simulink model "P702_NI_SoftECU"  (R2019a)
settings: Solver=ode1  StartTime=0.0  StopTime=Inf  FixedStep=0.001  RelTol=1e-3  EnableMultiTasking=on
PreLoadFcn:
  | run '.\VeriStand_BlockSet\NIVeriStandAddPaths.m'
undefined symbols (not defined in the file or in its folder): magnitude
libraries: simulink x83, simulink_extras x1
(part 75 of 76)

== system P702_NI_SoftECU/Output/Subsystem2/CAN_Signal/GWM/Other_GWMTx/Power_Liftgate_Stat_FD1 ==
  DrLckCnt_No_ActlTgate : Constant  Value=0
  DrTGate_D_Rq : Constant  Value=0
  DrTgateChime2_D_Rq : Constant  Value=0
  Power_Liftgate_Mode_Stt : Constant  Value=0
  PwLftgtIntSw_B_Stat : Constant  Value=0
  bus_creator : BusCreator  Inputs=5
  out_port : Outport
  wires:
  bus_creator/1 -> out_port/1  "Subsystem2"
  DrLckCnt_No_ActlTgate/1 -> bus_creator/1  "DrLckCnt_No_ActlTgate"
  DrTGate_D_Rq/1 -> bus_creator/2  "DrTGate_D_Rq"
  DrTgateChime2_D_Rq/1 -> bus_creator/3  "DrTgateChime2_D_Rq"
  Power_Liftgate_Mode_Stt/1 -> bus_creator/4  "Power_Liftgate_Mode_Stt"
  PwLftgtIntSw_B_Stat/1 -> bus_creator/5  "PwLftgtIntSw_B_Stat"

== system P702_NI_SoftECU/Output/Subsystem2/CAN_Signal/GWM/Other_GWMTx/PreCond_Hev_Data1_FD1 ==
  ChrgStat_D2_Dsply : Constant  Value=0
  bus_creator : BusCreator  Inputs=1
  out_port : Outport
  wires:
  bus_creator/1 -> out_port/1  "Subsystem2"
  ChrgStat_D2_Dsply/1 -> bus_creator/1  "ChrgStat_D2_Dsply"

== system P702_NI_SoftECU/Output/Subsystem2/CAN_Signal/GWM/Other_GWMTx/PreCond_Hev_Data2_FD1 ==
  BattTracClntFlw_Pc_Rq : Constant  Value=0
  BattTrac_I_EstVsc : Constant  Value=0
  DrvCondTpRrDefrs_B_Rq : Constant  Value=0
  HtrnAin_UHi_Actl : Constant  Value=0
  HtrnHvilOpen_B_Actl : Constant  Value=0
  HtrnMil_D_Rq : Constant  Value=0
  HtrnOvrTeLamp_B_Dsply : Constant  Value=0
  HtrnSrvcRqd_B_Dsply : Constant  Value=0
  PreCondActv_B_Actl : Constant  Value=0
  PtWakeupDeltaT_T_Rq : Constant  Value=0
  bus_creator : BusCreator  Inputs=10
  out_port : Outport
  wires:
  bus_creator/1 -> out_port/1  "Subsystem2"
  BattTracClntFlw_Pc_Rq/1 -> bus_creator/1  "BattTracClntFlw_Pc_Rq"
  BattTrac_I_EstVsc/1 -> bus_creator/2  "BattTrac_I_EstVsc"
  DrvCondTpRrDefrs_B_Rq/1 -> bus_creator/3  "DrvCondTpRrDefrs_B_Rq"
  HtrnAin_UHi_Actl/1 -> bus_creator/4  "HtrnAin_UHi_Actl"
  HtrnHvilOpen_B_Actl/1 -> bus_creator/5  "HtrnHvilOpen_B_Actl"
  HtrnMil_D_Rq/1 -> bus_creator/6  "HtrnMil_D_Rq"
  HtrnOvrTeLamp_B_Dsply/1 -> bus_creator/7  "HtrnOvrTeLamp_B_Dsply"
  HtrnSrvcRqd_B_Dsply/1 -> bus_creator/8  "HtrnSrvcRqd_B_Dsply"
  PreCondActv_B_Actl/1 -> bus_creator/9  "PreCondActv_B_Actl"
  PtWakeupDeltaT_T_Rq/1 -> bus_creator/10  "PtWakeupDeltaT_T_Rq"

== system P702_NI_SoftECU/Output/Subsystem2/CAN_Signal/GWM/Other_GWMTx/Suspension_Data_FD1 ==
  SuspClkSync_No_Rq : Constant  Value=0
  SuspFrntRight_L_Actl : Constant  Value=0
  SuspFrnt_L_Actl : Constant  Value=0
  SuspFrnt_L_Prev : Constant  Value=0
  SuspRearRight_L_Actl : Constant  Value=0
  SuspRear_L_Actl : Constant  Value=0
  SuspRear_L_Prev : Constant  Value=0
  bus_creator : BusCreator  Inputs=7
  out_port : Outport
  wires:
  bus_creator/1 -> out_port/1  "Subsystem2"
  SuspClkSync_No_Rq/1 -> bus_creator/1  "SuspClkSync_No_Rq"
  SuspFrntRight_L_Actl/1 -> bus_creator/2  "SuspFrntRight_L_Actl"
  SuspFrnt_L_Actl/1 -> bus_creator/3  "SuspFrnt_L_Actl"
  SuspFrnt_L_Prev/1 -> bus_creator/4  "SuspFrnt_L_Prev"
  SuspRearRight_L_Actl/1 -> bus_creator/5  "SuspRearRight_L_Actl"
  SuspRear_L_Actl/1 -> bus_creator/6  "SuspRear_L_Actl"
  SuspRear_L_Prev/1 -> bus_creator/7  "SuspRear_L_Prev"

== system P702_NI_SoftECU/Output/Subsystem2/CAN_Signal/GWM/Other_GWMTx/TesterPhysicalResGWM_FD1 ==
  TesterPhysicalResGWM_F1 : Constant  Value=0
  bus_creator : BusCreator  Inputs=1
  out_port : Outport
  wires:
  bus_creator/1 -> out_port/1  "Subsystem2"
  TesterPhysicalResGWM_F1/1 -> bus_creator/1  "TesterPhysicalResGWM_F1"

== system P702_NI_SoftECU/Output/Subsystem2/CAN_Signal/GWM/Other_GWMTx/TrailerAid_Data_FD1 ==
  TrlBrkInitOut_D_Rq : Constant  Value=0
  TrlrAidEnbl_D_Rq : Constant  Value=0
  TrlrAidSetup_D_Rq : Constant  Value=0
  TrlrAnOffstDir_D_Mem : Constant  Value=0
  TrlrAnOffst_An_Mem : Constant  Value=0
  TrlrAxleToBmpr_L_Actl : Constant  Value=0
  TrlrBallToBmpr_L_Actl : Constant  Value=0
  TrlrId_No_Actl : Constant  Value=0
  TrlrRvrseCancl_B_Rq : Constant  Value=0
  TrlrTrgtOffst_L_Actl : Constant  Value=0
  TrlrTrgtPtrnId_No_Mem : Constant  Value=0
  TrlrTrgtToBmpr_L_Actl : Constant  Value=0
  bus_creator : BusCreator  Inputs=12
  out_port : Outport
  wires:
  bus_creator/1 -> out_port/1  "Subsystem2"
  TrlBrkInitOut_D_Rq/1 -> bus_creator/1  "TrlBrkInitOut_D_Rq"
  TrlrAidEnbl_D_Rq/1 -> bus_creator/2  "TrlrAidEnbl_D_Rq"
  TrlrAidSetup_D_Rq/1 -> bus_creator/3  "TrlrAidSetup_D_Rq"
  TrlrAnOffstDir_D_Mem/1 -> bus_creator/4  "TrlrAnOffstDir_D_Mem"
  TrlrAnOffst_An_Mem/1 -> bus_creator/5  "TrlrAnOffst_An_Mem"
  TrlrAxleToBmpr_L_Actl/1 -> bus_creator/6  "TrlrAxleToBmpr_L_Actl"
  TrlrBallToBmpr_L_Actl/1 -> bus_creator/7  "TrlrBallToBmpr_L_Actl"
  TrlrId_No_Actl/1 -> bus_creator/8  "TrlrId_No_Actl"
  TrlrRvrseCancl_B_Rq/1 -> bus_creator/9  "TrlrRvrseCancl_B_Rq"
  TrlrTrgtOffst_L_Actl/1 -> bus_creator/10  "TrlrTrgtOffst_L_Actl"
  TrlrTrgtPtrnId_No_Mem/1 -> bus_creator/11  "TrlrTrgtPtrnId_No_Mem"
  TrlrTrgtToBmpr_L_Actl/1 -> bus_creator/12  "TrlrTrgtToBmpr_L_Actl"

== system P702_NI_SoftECU/Output/Subsystem2/CAN_Signal/GWM/Other_GWMTx/TrailerAid_Stat1_FD1 ==
  TrlrSnsId_No_Actl : Constant  Value=0
  bus_creator : BusCreator  Inputs=1
  out_port : Outport
  wires:
  bus_creator/1 -> out_port/1  "Subsystem2"
  TrlrSnsId_No_Actl/1 -> bus_creator/1  "TrlrSnsId_No_Actl"

== system P702_NI_SoftECU/Output/Subsystem2/CAN_Signal/GWM/Other_GWMTx/TrailerAid_Stat2_FD1 ==
  TrlrHitYaw_AnRate_Actl : Constant  Value=0
  TrlrHitchYaw_An_Actl : Constant  Value=0
  TrlrHitchYaw_D_Stat : Constant  Value=0
  TrlrYawWActl_D_Qf : Constant  Value=0
  TrlrYaw_W_Actl : Constant  Value=0
  bus_creator : BusCreator  Inputs=5
  out_port : Outport
  wires:
  bus_creator/1 -> out_port/1  "Subsystem2"
  TrlrHitYaw_AnRate_Actl/1 -> bus_creator/1  "TrlrHitYaw_AnRate_Actl"
  TrlrHitchYaw_An_Actl/1 -> bus_creator/2  "TrlrHitchYaw_An_Actl"
  TrlrHitchYaw_D_Stat/1 -> bus_creator/3  "TrlrHitchYaw_D_Stat"
  TrlrYawWActl_D_Qf/1 -> bus_creator/4  "TrlrYawWActl_D_Qf"
  TrlrYaw_W_Actl/1 -> bus_creator/5  "TrlrYaw_W_Actl"

== system P702_NI_SoftECU/Output/Subsystem2/CAN_Signal/GWM/Other_GWMTx/TrailerBrakeInfo_FD1 ==
  StopLamp_B_RqTrlrBrk : Constant  Value=0
  TrlBrkInitOut_D_Stat : Constant  Value=0
  TrlrBrkActCirct_B_Falt : Constant  Value=0
  TrlrBrkActCnnct_B_Actl : Constant  Value=0
  TrlrBrkCtl_B_Falt : Constant  Value=0
  TrlrBrkDcnnt_B_Actl : Constant  Value=0
  TrlrBrkDsply_B_Rq : Constant  Value=0
  TrlrBrkGain_No_Actl : Constant  Value=0
  TrlrBrkMde_D_Actl : Constant  Value=0
  TrlrBrkOut_No_Dsply : Constant  Value=0
  bus_creator : BusCreator  Inputs=10
  out_port : Outport
  wires:
  bus_creator/1 -> out_port/1  "Subsystem2"
  StopLamp_B_RqTrlrBrk/1 -> bus_creator/1  "StopLamp_B_RqTrlrBrk"
  TrlBrkInitOut_D_Stat/1 -> bus_creator/2  "TrlBrkInitOut_D_Stat"
  TrlrBrkActCirct_B_Falt/1 -> bus_creator/3  "TrlrBrkActCirct_B_Falt"
  TrlrBrkActCnnct_B_Actl/1 -> bus_creator/4  "TrlrBrkActCnnct_B_Actl"
  TrlrBrkCtl_B_Falt/1 -> bus_creator/5  "TrlrBrkCtl_B_Falt"
  TrlrBrkDcnnt_B_Actl/1 -> bus_creator/6  "TrlrBrkDcnnt_B_Actl"
  TrlrBrkDsply_B_Rq/1 -> bus_creator/7  "TrlrBrkDsply_B_Rq"
  TrlrBrkGain_No_Actl/1 -> bus_creator/8  "TrlrBrkGain_No_Actl"
  TrlrBrkMde_D_Actl/1 -> bus_creator/9  "TrlrBrkMde_D_Actl"
  TrlrBrkOut_No_Dsply/1 -> bus_creator/10  "TrlrBrkOut_No_Dsply"

== system P702_NI_SoftECU/Output/Subsystem2/CAN_Signal/GWM/Other_GWMTx/TrailerInfo_2_FD1 ==
  TrlrAidAn_URate_Actl : Constant  Value=0
  TrlrAidAn_U_Actl : Constant  Value=0
  TrlrAidCtl_U_RqDrv : Constant  Value=0
  TrlrAidSwtch_D_RqDrv : Constant  Value=0
  bus_creator : BusCreator  Inputs=4
  out_port : Outport
  wires:
  bus_creator/1 -> out_port/1  "Subsystem2"
  TrlrAidAn_URate_Actl/1 -> bus_creator/1  "TrlrAidAn_URate_Actl"
  TrlrAidAn_U_Actl/1 -> bus_creator/2  "TrlrAidAn_U_Actl"
  TrlrAidCtl_U_RqDrv/1 -> bus_creator/3  "TrlrAidCtl_U_RqDrv"
  TrlrAidSwtch_D_RqDrv/1 -> bus_creator/4  "TrlrAidSwtch_D_RqDrv"

== system P702_NI_SoftECU/Output/Subsystem2/CAN_Signal/GWM/Other_GWMTx/TrailerInfo_FD1 ==
  ParkLampTrlrOut_B_Stat : Constant  Value=0
  StopLampTrlrOut_B_Stat : Constant  Value=0
  TrlrBattChrg_D_Stat : Constant  Value=0
  TrlrLampCnnct_B_Actl : Constant  Value=0
  TrlrLampCtl_D_Stat : Constant  Value=0
  TurnLampTrlrRl_B_Stat : Constant  Value=0
  TurnLampTrlrRr_B_Stat : Constant  Value=0
  bus_creator : BusCreator  Inputs=7
  out_port : Outport
  wires:
  bus_creator/1 -> out_port/1  "Subsystem2"
  ParkLampTrlrOut_B_Stat/1 -> bus_creator/1  "ParkLampTrlrOut_B_Stat"
  StopLampTrlrOut_B_Stat/1 -> bus_creator/2  "StopLampTrlrOut_B_Stat"
  TrlrBattChrg_D_Stat/1 -> bus_creator/3  "TrlrBattChrg_D_Stat"
  TrlrLampCnnct_B_Actl/1 -> bus_creator/4  "TrlrLampCnnct_B_Actl"
  TrlrLampCtl_D_Stat/1 -> bus_creator/5  "TrlrLampCtl_D_Stat"
  TurnLampTrlrRl_B_Stat/1 -> bus_creator/6  "TurnLampTrlrRl_B_Stat"
  TurnLampTrlrRr_B_Stat/1 -> bus_creator/7  "TurnLampTrlrRr_B_Stat"

== system P702_NI_SoftECU/Output/Subsystem2/CAN_Signal/GWM/Other_GWMTx/VeyDynamics_Data_FD1 ==
  AdptDrvMdeChassis_D_Rq : Constant  Value=0
  AdptDrvMdePt_D_Rq : Constant  Value=0
  AirSprngRateFl_D_Rq : Constant  Value=0
  AirSprngRateFr_D_Rq : Constant  Value=0
  AirSprngRateRl_D_Rq : Constant  Value=0
  AirSprngRateRr_D_Rq : Constant  Value=0
  AirSuspMsgTxt_D_Rq : Constant  Value=0
  AirSusp_D_Stat : Constant  Value=0
  BrkPadMsgTxt_D_Rq : Constant  Value=0
  CcdMsgTxt_D_RqDsply : Constant  Value=0
  Ccd_B_Falt : Constant  Value=0
  SelDrvMdeSusp_D_Stat : Constant  Value=0
  SuspDrvMde_D_Stat : Constant  Value=0
  SuspType_B_Stat : Constant  Value=0
  SuspVLim_B_Rq : Constant  Value=0
  bus_creator : BusCreator  Inputs=15
  out_port : Outport
  wires:
  bus_creator/1 -> out_port/1  "Subsystem2"
  AdptDrvMdeChassis_D_Rq/1 -> bus_creator/1  "AdptDrvMdeChassis_D_Rq"
  AdptDrvMdePt_D_Rq/1 -> bus_creator/2  "AdptDrvMdePt_D_Rq"
  AirSprngRateFl_D_Rq/1 -> bus_creator/3  "AirSprngRateFl_D_Rq"
  AirSprngRateFr_D_Rq/1 -> bus_creator/4  "AirSprngRateFr_D_Rq"
  AirSprngRateRl_D_Rq/1 -> bus_creator/5  "AirSprngRateRl_D_Rq"
  AirSprngRateRr_D_Rq/1 -> bus_creator/6  "AirSprngRateRr_D_Rq"
  AirSuspMsgTxt_D_Rq/1 -> bus_creator/7  "AirSuspMsgTxt_D_Rq"
  AirSusp_D_Stat/1 -> bus_creator/8  "AirSusp_D_Stat"
  BrkPadMsgTxt_D_Rq/1 -> bus_creator/9  "BrkPadMsgTxt_D_Rq"
  CcdMsgTxt_D_RqDsply/1 -> bus_creator/10  "CcdMsgTxt_D_RqDsply"
  Ccd_B_Falt/1 -> bus_creator/11  "Ccd_B_Falt"
  SelDrvMdeSusp_D_Stat/1 -> bus_creator/12  "SelDrvMdeSusp_D_Stat"
  SuspDrvMde_D_Stat/1 -> bus_creator/13  "SuspDrvMde_D_Stat"
  SuspType_B_Stat/1 -> bus_creator/14  "SuspType_B_Stat"
  SuspVLim_B_Rq/1 -> bus_creator/15  "SuspVLim_B_Rq"

== system P702_NI_SoftECU/Output/Subsystem2/CAN_Signal/GWM/RCM/RCMSerialNumber_FD1_454 ==
  RCMSerialNoByte{1..8} (8 alike) : Constant  Value=0
  bus_creator : BusCreator  Inputs=8
  out_port : Outport
  wires:
  bus_creator/1 -> out_port/1  "Subsystem2"
  RCMSerialNoByte1/1 -> bus_creator/1  "RCMSerialNoByte1"
  RCMSerialNoByte2/1 -> bus_creator/2  "RCMSerialNoByte2"
  RCMSerialNoByte3/1 -> bus_creator/3  "RCMSerialNoByte3"
  RCMSerialNoByte4/1 -> bus_creator/4  "RCMSerialNoByte4"
  RCMSerialNoByte5/1 -> bus_creator/5  "RCMSerialNoByte5"
  RCMSerialNoByte6/1 -> bus_creator/6  "RCMSerialNoByte6"
  RCMSerialNoByte7/1 -> bus_creator/7  "RCMSerialNoByte7"
  RCMSerialNoByte8/1 -> bus_creator/8  "RCMSerialNoByte8"

== system P702_NI_SoftECU/Output/Subsystem2/CAN_Signal/GWM/RCM/RCMStatusMessage2_FD1_4C ==
  EDRTriggerEvntSync : Constant  Value=0
  FirstRowBuckleDriver : Constant  Value=0
  FirstRowBuckleMid : Constant  Value=0
  FirstRowBucklePsngr : Constant  Value=0
  PassRstrnInd_Req : Constant  Value=0
  PsngrFmidDetct_D_Actl : Constant  Value=0
  PsngrFrntDetct_D_Actl : Constant  Value=0
  RILReq : Constant  Value=0
  RstrnImpactEvntStatus : Constant  Value=0
  RstrnPsngrOn_D_Stat : Constant  Value=0
  SecondRowBuckleDriver : Constant  Value=0
  SecondRowBuckleMid : Constant  Value=0
  SecondRowBucklePsngr : Constant  Value=0
  ThirdRowBuckleDriver : Constant  Value=0
  ThirdRowBuckleMid : Constant  Value=0
  ThirdRowBucklePsngr : Constant  Value=0
  bus_creator : BusCreator  Inputs=16
  out_port : Outport
  wires:
  bus_creator/1 -> out_port/1  "Subsystem2"
  EDRTriggerEvntSync/1 -> bus_creator/1  "EDRTriggerEvntSync"
  FirstRowBuckleDriver/1 -> bus_creator/2  "FirstRowBuckleDriver"
  FirstRowBuckleMid/1 -> bus_creator/3  "FirstRowBuckleMid"
  FirstRowBucklePsngr/1 -> bus_creator/4  "FirstRowBucklePsngr"
  PassRstrnInd_Req/1 -> bus_creator/5  "PassRstrnInd_Req"
  PsngrFmidDetct_D_Actl/1 -> bus_creator/6  "PsngrFmidDetct_D_Actl"
  PsngrFrntDetct_D_Actl/1 -> bus_creator/7  "PsngrFrntDetct_D_Actl"
  RILReq/1 -> bus_creator/8  "RILReq"
  RstrnImpactEvntStatus/1 -> bus_creator/9  "RstrnImpactEvntStatus"
  RstrnPsngrOn_D_Stat/1 -> bus_creator/10  "RstrnPsngrOn_D_Stat"
  SecondRowBuckleDriver/1 -> bus_creator/11  "SecondRowBuckleDriver"
  SecondRowBuckleMid/1 -> bus_creator/12  "SecondRowBuckleMid"
  SecondRowBucklePsngr/1 -> bus_creator/13  "SecondRowBucklePsngr"
  ThirdRowBuckleDriver/1 -> bus_creator/14  "ThirdRowBuckleDriver"
  ThirdRowBuckleMid/1 -> bus_creator/15  "ThirdRowBuckleMid"
  ThirdRowBucklePsngr/1 -> bus_creator/16  "ThirdRowBucklePsngr"

== system P702_NI_SoftECU/Output/Subsystem2/CAN_Signal/GWM/SCCM/Steering_Data_FD1_83 ==
  AccButtnGapDecPress : Constant  Value=0
  AccButtnGapIncPress : Constant  Value=0
  AccButtnGapTogglePress : Constant  Value=0
  AhbStat_B_Dsply : Constant  Value=0
  AslButtnOnOffCnclPress : Constant  Value=0
  AslButtnOnOffPress : Constant  Value=0
  CcAslButtnCnclPress : Constant  Value=0
  CcAslButtnCnclResPress : Constant  Value=0
  CcAslButtnDeny_B_Actl : Constant  Value=0
  CcAslButtnIndxDecPress : Constant  Value=0
  CcAslButtnIndxIncPress : Constant  Value=0
  CcAslButtnOffCnclPress : Constant  Value=0
  CcAslButtnOnOffCncl : Constant  Value=0
  CcAslButtnOnPress : Constant  Value=0
  CcAslButtnResDecPress : Constant  Value=0
  CcAslButtnResIncPress : Constant  Value=0
  CcAslButtnSetDecPress : Constant  Value=0
  CcAslButtnSetIncPress : Constant  Value=0
  CcAslButtnSetPress : Constant  Value=0
  CcAsllButtnResPress : Constant  Value=0
  CcButtnOffPress : Constant  Value=0
  CcButtnOnOffCnclPress : Constant  Value=0
  CcButtnOnOffPress : Constant  Value=0
  CcButtnOnPress : Constant  Value=0
  HeadLghtHiCtrl_D_RqAhb : Constant  Value=0
  HeadLghtHiFlash_D_Actl : Constant  Value=0
  HeadLghtHiFlash_D_Stat : Constant  Value=0
  HeadLghtHiOn_B_StatAhb : Constant  Value=0
  LaSwtchPos_D_Stat : Constant  Value=0
  LghtAmb_D_Sns : Constant  Value=0
  TjaButtnOnOffPress : Constant  Value=0
  TurnLghtSwtch_D_Stat : Constant  Value=0
  WiprFrontSwtch_D_Stat : Constant  Value=0
  WiprFront_D_Stat : Constant  Value=0
  bus_creator : BusCreator  Inputs=34
  out_port : Outport
  wires:
  bus_creator/1 -> out_port/1  "Subsystem2"
  AccButtnGapDecPress/1 -> bus_creator/1  "AccButtnGapDecPress"
  AccButtnGapIncPress/1 -> bus_creator/2  "AccButtnGapIncPress"
  AccButtnGapTogglePress/1 -> bus_creator/3  "AccButtnGapTogglePress"
  AhbStat_B_Dsply/1 -> bus_creator/4  "AhbStat_B_Dsply"
  AslButtnOnOffCnclPress/1 -> bus_creator/5  "AslButtnOnOffCnclPress"
  AslButtnOnOffPress/1 -> bus_creator/6  "AslButtnOnOffPress"
  CcAslButtnCnclPress/1 -> bus_creator/7  "CcAslButtnCnclPress"
  CcAslButtnCnclResPress/1 -> bus_creator/8  "CcAslButtnCnclResPress"
  CcAslButtnDeny_B_Actl/1 -> bus_creator/9  "CcAslButtnDeny_B_Actl"
  CcAslButtnIndxDecPress/1 -> bus_creator/10  "CcAslButtnIndxDecPress"
  CcAslButtnIndxIncPress/1 -> bus_creator/11  "CcAslButtnIndxIncPress"
  CcAslButtnOffCnclPress/1 -> bus_creator/12  "CcAslButtnOffCnclPress"
  CcAslButtnOnOffCncl/1 -> bus_creator/13  "CcAslButtnOnOffCncl"
  CcAslButtnOnPress/1 -> bus_creator/14  "CcAslButtnOnPress"
  CcAslButtnResDecPress/1 -> bus_creator/15  "CcAslButtnResDecPress"
  CcAslButtnResIncPress/1 -> bus_creator/16  "CcAslButtnResIncPress"
  CcAslButtnSetDecPress/1 -> bus_creator/17  "CcAslButtnSetDecPress"
  CcAslButtnSetIncPress/1 -> bus_creator/18  "CcAslButtnSetIncPress"
  CcAslButtnSetPress/1 -> bus_creator/19  "CcAslButtnSetPress"
  CcAsllButtnResPress/1 -> bus_creator/20  "CcAsllButtnResPress"
  CcButtnOffPress/1 -> bus_creator/21  "CcButtnOffPress"
  CcButtnOnOffCnclPress/1 -> bus_creator/22  "CcButtnOnOffCnclPress"
  CcButtnOnOffPress/1 -> bus_creator/23  "CcButtnOnOffPress"
  CcButtnOnPress/1 -> bus_creator/24  "CcButtnOnPress"
  HeadLghtHiCtrl_D_RqAhb/1 -> bus_creator/25  "HeadLghtHiCtrl_D_RqAhb"
  HeadLghtHiFlash_D_Actl/1 -> bus_creator/26  "HeadLghtHiFlash_D_Actl"
  HeadLghtHiFlash_D_Stat/1 -> bus_creator/27  "HeadLghtHiFlash_D_Stat"
  HeadLghtHiOn_B_StatAhb/1 -> bus_creator/28  "HeadLghtHiOn_B_StatAhb"
  LaSwtchPos_D_Stat/1 -> bus_creator/29  "LaSwtchPos_D_Stat"
  LghtAmb_D_Sns/1 -> bus_creator/30  "LghtAmb_D_Sns"
  TjaButtnOnOffPress/1 -> bus_creator/31  "TjaButtnOnOffPress"
  TurnLghtSwtch_D_Stat/1 -> bus_creator/32  "TurnLghtSwtch_D_Stat"
  WiprFrontSwtch_D_Stat/1 -> bus_creator/33  "WiprFrontSwtch_D_Stat"
  WiprFront_D_Stat/1 -> bus_creator/34  "WiprFront_D_Stat"

== system P702_NI_SoftECU/Output/Subsystem2/CAN_Signal/GWM/SCCM/Steering_Wheel_Data2_FD1_81 ==
  SelDrvMdeDec_B_RqDrv : Constant  Value=0
  SelDrvMdeInc_B_RqDrv : Constant  Value=0
  SelDrvMdeSwtch_D_Stat4 : Constant  Value=0
  SteEffortInc_B_RqDrv : Constant  Value=0
  SteWhlSwtchBack_B_Stat : Constant  Value=0
  SteWhlSwtchDown_B_Stat : Constant  Value=0
  SteWhlSwtchHome_B_Stat : Constant  Value=0
  SteWhlSwtchHud_B_Stat : Constant  Value=0
  SteWhlSwtchInfo_B_Stat : Constant  Value=0
  SteWhlSwtchIod_B_Stat : Constant  Value=0
  SteWhlSwtchLeft_B_Stat : Constant  Value=0
  SteWhlSwtchMed_B_Stat : Constant  Value=0
  SteWhlSwtchMenu_B_Stat : Constant  Value=0
  SteWhlSwtchNav_B_Stat : Constant  Value=0
  SteWhlSwtchOk_B_Stat : Constant  Value=0
  SteWhlSwtchPhon_B_Stat : Constant  Value=0
  SteWhlSwtchRght_B_Stat : Constant  Value=0
  SteWhlSwtchSet_B_Stat : Constant  Value=0
  SteWhlSwtchUp_B_Stat : Constant  Value=0
  SteWhlSwtchView_B_Stat : Constant  Value=0
  SuspDampInc_B_RqDrv : Constant  Value=0
  bus_creator : BusCreator  Inputs=21
  out_port : Outport
  wires:
  bus_creator/1 -> out_port/1  "Subsystem2"
  SelDrvMdeDec_B_RqDrv/1 -> bus_creator/1  "SelDrvMdeDec_B_RqDrv"
  SelDrvMdeInc_B_RqDrv/1 -> bus_creator/2  "SelDrvMdeInc_B_RqDrv"
  SelDrvMdeSwtch_D_Stat4/1 -> bus_creator/3  "SelDrvMdeSwtch_D_Stat4"
  SteEffortInc_B_RqDrv/1 -> bus_creator/4  "SteEffortInc_B_RqDrv"
  SteWhlSwtchBack_B_Stat/1 -> bus_creator/5  "SteWhlSwtchBack_B_Stat"
  SteWhlSwtchDown_B_Stat/1 -> bus_creator/6  "SteWhlSwtchDown_B_Stat"
  SteWhlSwtchHome_B_Stat/1 -> bus_creator/7  "SteWhlSwtchHome_B_Stat"
  SteWhlSwtchHud_B_Stat/1 -> bus_creator/8  "SteWhlSwtchHud_B_Stat"
  SteWhlSwtchInfo_B_Stat/1 -> bus_creator/9  "SteWhlSwtchInfo_B_Stat"
  SteWhlSwtchIod_B_Stat/1 -> bus_creator/10  "SteWhlSwtchIod_B_Stat"
  SteWhlSwtchLeft_B_Stat/1 -> bus_creator/11  "SteWhlSwtchLeft_B_Stat"
  SteWhlSwtchMed_B_Stat/1 -> bus_creator/12  "SteWhlSwtchMed_B_Stat"
  SteWhlSwtchMenu_B_Stat/1 -> bus_creator/13  "SteWhlSwtchMenu_B_Stat"
  SteWhlSwtchNav_B_Stat/1 -> bus_creator/14  "SteWhlSwtchNav_B_Stat"
  SteWhlSwtchOk_B_Stat/1 -> bus_creator/15  "SteWhlSwtchOk_B_Stat"
  SteWhlSwtchPhon_B_Stat/1 -> bus_creator/16  "SteWhlSwtchPhon_B_Stat"
  SteWhlSwtchRght_B_Stat/1 -> bus_creator/17  "SteWhlSwtchRght_B_Stat"
  SteWhlSwtchSet_B_Stat/1 -> bus_creator/18  "SteWhlSwtchSet_B_Stat"
  SteWhlSwtchUp_B_Stat/1 -> bus_creator/19  "SteWhlSwtchUp_B_Stat"
  SteWhlSwtchView_B_Stat/1 -> bus_creator/20  "SteWhlSwtchView_B_Stat"
  SuspDampInc_B_RqDrv/1 -> bus_creator/21  "SuspDampInc_B_RqDrv"

== system P702_NI_SoftECU/Output/Subsystem2/CAN_Signal/GWM/Tester//AutoSar/GWM_AutoSar_NetMgmt_FD1 ==
  GWM_AutoSarNMControl : Constant  Value=0
  GWM_AutoSarNMNodeId : Constant  Value=0
  GWM_AutoSarNMReserved{1..4} (4 alike) : Constant  Value=0
  GWM_GWNMProxy : Constant  Value=0
  GWM_GWOnBoardTester : Constant  Value=0
  bus_creator : BusCreator  Inputs=8
  out_port : Outport
  wires:
  bus_creator/1 -> out_port/1  "Subsystem2"
  GWM_AutoSarNMControl/1 -> bus_creator/1  "GWM_AutoSarNMControl"
  GWM_AutoSarNMNodeId/1 -> bus_creator/2  "GWM_AutoSarNMNodeId"
  GWM_AutoSarNMReserved1/1 -> bus_creator/3  "GWM_AutoSarNMReserved1"
  GWM_AutoSarNMReserved2/1 -> bus_creator/4  "GWM_AutoSarNMReserved2"
  GWM_AutoSarNMReserved3/1 -> bus_creator/5  "GWM_AutoSarNMReserved3"
  GWM_AutoSarNMReserved4/1 -> bus_creator/6  "GWM_AutoSarNMReserved4"
  GWM_GWNMProxy/1 -> bus_creator/7  "GWM_GWNMProxy"
  GWM_GWOnBoardTester/1 -> bus_creator/8  "GWM_GWOnBoardTester"

== system P702_NI_SoftECU/Output/Subsystem2/CAN_Signal/GWM/Tester//AutoSar/TesterPhysicalResGWM_FD1 ==
  TesterPhysicalResGWM_F1 : Constant  Value=0
  bus_creator : BusCreator  Inputs=1
  out_port : Outport
  wires:
  bus_creator/1 -> out_port/1  "Subsystem2"
  TesterPhysicalResGWM_F1/1 -> bus_creator/1  "TesterPhysicalResGWM_F1"

== system P702_NI_SoftECU/Output/Subsystem2/To_NI_HIL/SRR_L/FL_SOD/SRR_FL_001 ==
  SRR_FL_CAN_DET_AMPLITUDE_01 : Constant  Value=0
  SRR_FL_CAN_DET_AZIMUTH_01 : Constant  Value=0
  SRR_FL_CAN_DET_ELEVATION_01 : Constant  Value=0
  SRR_FL_CAN_DET_RANGE_01 : Constant  Value=0
  SRR_FL_CAN_DET_RANGE_RATE_01 : Constant  Value=0
  SRR_FL_CAN_DET_SUPER_RES_TARGET_01 : Constant  Value=0
  SRR_FL_CAN_DET_VALID_LEVEL_01 : Constant  Value=0
  bus_creator : BusCreator  Inputs=7
  out_port : Outport
  wires:
  bus_creator/1 -> out_port/1  "Subsystem2"
  SRR_FL_CAN_DET_RANGE_01/1 -> bus_creator/1  "SRR_FL_CAN_DET_RANGE_01"
  SRR_FL_CAN_DET_RANGE_RATE_01/1 -> bus_creator/2  "SRR_FL_CAN_DET_RANGE_RATE_01"
  SRR_FL_CAN_DET_AZIMUTH_01/1 -> bus_creator/3  "SRR_FL_CAN_DET_AZIMUTH_01"
  SRR_FL_CAN_DET_ELEVATION_01/1 -> bus_creator/4  "SRR_FL_CAN_DET_ELEVATION_01"
  SRR_FL_CAN_DET_SUPER_RES_TARGET_01/1 -> bus_creator/5  "SRR_FL_CAN_DET_SUPER_RES_TARGET_01"
  SRR_FL_CAN_DET_AMPLITUDE_01/1 -> bus_creator/6  "SRR_FL_CAN_DET_AMPLITUDE_01"
  SRR_FL_CAN_DET_VALID_LEVEL_01/1 -> bus_creator/7  "SRR_FL_CAN_DET_VALID_LEVEL_01"

== system P702_NI_SoftECU/Output/Subsystem2/To_NI_HIL/SRR_L/FL_SOD/SRR_FL_002 ==
  SRR_FL_CAN_DET_AMPLITUDE_02 : Constant  Value=0
  SRR_FL_CAN_DET_AZIMUTH_02 : Constant  Value=0
  SRR_FL_CAN_DET_ELEVATION_02 : Constant  Value=0
  SRR_FL_CAN_DET_RANGE_02 : Constant  Value=0
  SRR_FL_CAN_DET_RANGE_RATE_02 : Constant  Value=0
  SRR_FL_CAN_DET_SUPER_RES_TARGET_02 : Constant  Value=0
  SRR_FL_CAN_DET_VALID_LEVEL_02 : Constant  Value=0
  bus_creator : BusCreator  Inputs=7
  out_port : Outport
  wires:
  bus_creator/1 -> out_port/1  "Subsystem2"
  SRR_FL_CAN_DET_RANGE_02/1 -> bus_creator/1  "SRR_FL_CAN_DET_RANGE_02"
  SRR_FL_CAN_DET_RANGE_RATE_02/1 -> bus_creator/2  "SRR_FL_CAN_DET_RANGE_RATE_02"
  SRR_FL_CAN_DET_AZIMUTH_02/1 -> bus_creator/3  "SRR_FL_CAN_DET_AZIMUTH_02"
  SRR_FL_CAN_DET_ELEVATION_02/1 -> bus_creator/4  "SRR_FL_CAN_DET_ELEVATION_02"
  SRR_FL_CAN_DET_SUPER_RES_TARGET_02/1 -> bus_creator/5  "SRR_FL_CAN_DET_SUPER_RES_TARGET_02"
  SRR_FL_CAN_DET_AMPLITUDE_02/1 -> bus_creator/6  "SRR_FL_CAN_DET_AMPLITUDE_02"
  SRR_FL_CAN_DET_VALID_LEVEL_02/1 -> bus_creator/7  "SRR_FL_CAN_DET_VALID_LEVEL_02"

== system P702_NI_SoftECU/Output/Subsystem2/To_NI_HIL/SRR_L/FL_SOD/SRR_FL_003 ==
  SRR_FL_CAN_DET_AMPLITUDE_03 : Constant  Value=0
  SRR_FL_CAN_DET_AZIMUTH_03 : Constant  Value=0
  SRR_FL_CAN_DET_ELEVATION_03 : Constant  Value=0
  SRR_FL_CAN_DET_RANGE_03 : Constant  Value=0
  SRR_FL_CAN_DET_RANGE_RATE_03 : Constant  Value=0
  SRR_FL_CAN_DET_SUPER_RES_TARGET_03 : Constant  Value=0
  SRR_FL_CAN_DET_VALID_LEVEL_03 : Constant  Value=0
  bus_creator : BusCreator  Inputs=7
  out_port : Outport
  wires:
  bus_creator/1 -> out_port/1  "Subsystem2"
  SRR_FL_CAN_DET_RANGE_03/1 -> bus_creator/1  "SRR_FL_CAN_DET_RANGE_03"
  SRR_FL_CAN_DET_RANGE_RATE_03/1 -> bus_creator/2  "SRR_FL_CAN_DET_RANGE_RATE_03"
  SRR_FL_CAN_DET_AZIMUTH_03/1 -> bus_creator/3  "SRR_FL_CAN_DET_AZIMUTH_03"
  SRR_FL_CAN_DET_ELEVATION_03/1 -> bus_creator/4  "SRR_FL_CAN_DET_ELEVATION_03"
  SRR_FL_CAN_DET_SUPER_RES_TARGET_03/1 -> bus_creator/5  "SRR_FL_CAN_DET_SUPER_RES_TARGET_03"
  SRR_FL_CAN_DET_AMPLITUDE_03/1 -> bus_creator/6  "SRR_FL_CAN_DET_AMPLITUDE_03"
  SRR_FL_CAN_DET_VALID_LEVEL_03/1 -> bus_creator/7  "SRR_FL_CAN_DET_VALID_LEVEL_03"

== system P702_NI_SoftECU/Output/Subsystem2/To_NI_HIL/SRR_L/RL_SOD/SRR_RL_001 ==
  SRR_RL_CAN_DET_AMPLITUDE_01 : Constant  Value=0
  SRR_RL_CAN_DET_AZIMUTH_01 : Constant  Value=0
  SRR_RL_CAN_DET_ELEVATION_01 : Constant  Value=0
  SRR_RL_CAN_DET_RANGE_01 : Constant  Value=0
  SRR_RL_CAN_DET_RANGE_RATE_01 : Constant  Value=0
  SRR_RL_CAN_DET_SUPER_RES_TARGET_01 : Constant  Value=0
  SRR_RL_CAN_DET_VALID_LEVEL_01 : Constant  Value=0
  bus_creator : BusCreator  Inputs=7
  out_port : Outport
  wires:
  bus_creator/1 -> out_port/1  "Subsystem2"
  SRR_RL_CAN_DET_RANGE_01/1 -> bus_creator/1  "SRR_RL_CAN_DET_RANGE_01"
  SRR_RL_CAN_DET_RANGE_RATE_01/1 -> bus_creator/2  "SRR_RL_CAN_DET_RANGE_RATE_01"
  SRR_RL_CAN_DET_AZIMUTH_01/1 -> bus_creator/3  "SRR_RL_CAN_DET_AZIMUTH_01"
  SRR_RL_CAN_DET_ELEVATION_01/1 -> bus_creator/4  "SRR_RL_CAN_DET_ELEVATION_01"
  SRR_RL_CAN_DET_SUPER_RES_TARGET_01/1 -> bus_creator/5  "SRR_RL_CAN_DET_SUPER_RES_TARGET_01"
  SRR_RL_CAN_DET_AMPLITUDE_01/1 -> bus_creator/6  "SRR_RL_CAN_DET_AMPLITUDE_01"
  SRR_RL_CAN_DET_VALID_LEVEL_01/1 -> bus_creator/7  "SRR_RL_CAN_DET_VALID_LEVEL_01"

== system P702_NI_SoftECU/Output/Subsystem2/To_NI_HIL/SRR_L/RL_SOD/SRR_RL_002 ==
  SRR_RL_CAN_DET_AMPLITUDE_02 : Constant  Value=0
  SRR_RL_CAN_DET_AZIMUTH_02 : Constant  Value=0
  SRR_RL_CAN_DET_ELEVATION_02 : Constant  Value=0
  SRR_RL_CAN_DET_RANGE_02 : Constant  Value=0
  SRR_RL_CAN_DET_RANGE_RATE_02 : Constant  Value=0
  SRR_RL_CAN_DET_SUPER_RES_TARGET_02 : Constant  Value=0
  SRR_RL_CAN_DET_VALID_LEVEL_02 : Constant  Value=0
  bus_creator : BusCreator  Inputs=7
  out_port : Outport
  wires:
  bus_creator/1 -> out_port/1  "Subsystem2"
  SRR_RL_CAN_DET_RANGE_02/1 -> bus_creator/1  "SRR_RL_CAN_DET_RANGE_02"
  SRR_RL_CAN_DET_RANGE_RATE_02/1 -> bus_creator/2  "SRR_RL_CAN_DET_RANGE_RATE_02"
  SRR_RL_CAN_DET_AZIMUTH_02/1 -> bus_creator/3  "SRR_RL_CAN_DET_AZIMUTH_02"
  SRR_RL_CAN_DET_ELEVATION_02/1 -> bus_creator/4  "SRR_RL_CAN_DET_ELEVATION_02"
  SRR_RL_CAN_DET_SUPER_RES_TARGET_02/1 -> bus_creator/5  "SRR_RL_CAN_DET_SUPER_RES_TARGET_02"
  SRR_RL_CAN_DET_AMPLITUDE_02/1 -> bus_creator/6  "SRR_RL_CAN_DET_AMPLITUDE_02"
  SRR_RL_CAN_DET_VALID_LEVEL_02/1 -> bus_creator/7  "SRR_RL_CAN_DET_VALID_LEVEL_02"

== system P702_NI_SoftECU/Output/Subsystem2/To_NI_HIL/SRR_L/RL_SOD/SRR_RL_003 ==
  SRR_RL_CAN_DET_AMPLITUDE_03 : Constant  Value=0
  SRR_RL_CAN_DET_AZIMUTH_03 : Constant  Value=0
  SRR_RL_CAN_DET_ELEVATION_03 : Constant  Value=0
  SRR_RL_CAN_DET_RANGE_03 : Constant  Value=0
  SRR_RL_CAN_DET_RANGE_RATE_03 : Constant  Value=0
  SRR_RL_CAN_DET_SUPER_RES_TARGET_03 : Constant  Value=0
  SRR_RL_CAN_DET_VALID_LEVEL_03 : Constant  Value=0
  bus_creator : BusCreator  Inputs=7
  out_port : Outport
  wires:
  bus_creator/1 -> out_port/1  "Subsystem2"
  SRR_RL_CAN_DET_RANGE_03/1 -> bus_creator/1  "SRR_RL_CAN_DET_RANGE_03"
  SRR_RL_CAN_DET_RANGE_RATE_03/1 -> bus_creator/2  "SRR_RL_CAN_DET_RANGE_RATE_03"
  SRR_RL_CAN_DET_AZIMUTH_03/1 -> bus_creator/3  "SRR_RL_CAN_DET_AZIMUTH_03"
  SRR_RL_CAN_DET_ELEVATION_03/1 -> bus_creator/4  "SRR_RL_CAN_DET_ELEVATION_03"
  SRR_RL_CAN_DET_SUPER_RES_TARGET_03/1 -> bus_creator/5  "SRR_RL_CAN_DET_SUPER_RES_TARGET_03"
  SRR_RL_CAN_DET_AMPLITUDE_03/1 -> bus_creator/6  "SRR_RL_CAN_DET_AMPLITUDE_03"
  SRR_RL_CAN_DET_VALID_LEVEL_03/1 -> bus_creator/7  "SRR_RL_CAN_DET_VALID_LEVEL_03"

== system P702_NI_SoftECU/Output/Subsystem2/To_NI_HIL/SRR_R/FR_SOD/SRR_FR_001 ==
  SRR_FR_CAN_DET_AMPLITUDE_01 : Constant  Value=0
  SRR_FR_CAN_DET_AZIMUTH_01 : Constant  Value=0
  SRR_FR_CAN_DET_ELEVATION_01 : Constant  Value=0
  SRR_FR_CAN_DET_RANGE_01 : Constant  Value=0
  SRR_FR_CAN_DET_RANGE_RATE_01 : Constant  Value=0
  SRR_FR_CAN_DET_SUPER_RES_TARGET_01 : Constant  Value=0
  SRR_FR_CAN_DET_VALID_LEVEL_01 : Constant  Value=0
  bus_creator : BusCreator  Inputs=7
  out_port : Outport
  wires:
  bus_creator/1 -> out_port/1  "Subsystem2"
  SRR_FR_CAN_DET_RANGE_01/1 -> bus_creator/1  "SRR_FR_CAN_DET_RANGE_01"
  SRR_FR_CAN_DET_RANGE_RATE_01/1 -> bus_creator/2  "SRR_FR_CAN_DET_RANGE_RATE_01"
  SRR_FR_CAN_DET_AZIMUTH_01/1 -> bus_creator/3  "SRR_FR_CAN_DET_AZIMUTH_01"
  SRR_FR_CAN_DET_ELEVATION_01/1 -> bus_creator/4  "SRR_FR_CAN_DET_ELEVATION_01"
  SRR_FR_CAN_DET_SUPER_RES_TARGET_01/1 -> bus_creator/5  "SRR_FR_CAN_DET_SUPER_RES_TARGET_01"
  SRR_FR_CAN_DET_AMPLITUDE_01/1 -> bus_creator/6  "SRR_FR_CAN_DET_AMPLITUDE_01"
  SRR_FR_CAN_DET_VALID_LEVEL_01/1 -> bus_creator/7  "SRR_FR_CAN_DET_VALID_LEVEL_01"

== system P702_NI_SoftECU/Output/Subsystem2/To_NI_HIL/SRR_R/FR_SOD/SRR_FR_002 ==
  SRR_FR_CAN_DET_AMPLITUDE_02 : Constant  Value=0
  SRR_FR_CAN_DET_AZIMUTH_02 : Constant  Value=0
  SRR_FR_CAN_DET_ELEVATION_02 : Constant  Value=0
  SRR_FR_CAN_DET_RANGE_02 : Constant  Value=0
  SRR_FR_CAN_DET_RANGE_RATE_02 : Constant  Value=0
  SRR_FR_CAN_DET_SUPER_RES_TARGET_02 : Constant  Value=0
  SRR_FR_CAN_DET_VALID_LEVEL_02 : Constant  Value=0
  bus_creator : BusCreator  Inputs=7
  out_port : Outport
  wires:
  bus_creator/1 -> out_port/1  "Subsystem2"
  SRR_FR_CAN_DET_RANGE_02/1 -> bus_creator/1  "SRR_FR_CAN_DET_RANGE_02"
  SRR_FR_CAN_DET_RANGE_RATE_02/1 -> bus_creator/2  "SRR_FR_CAN_DET_RANGE_RATE_02"
  SRR_FR_CAN_DET_AZIMUTH_02/1 -> bus_creator/3  "SRR_FR_CAN_DET_AZIMUTH_02"
  SRR_FR_CAN_DET_ELEVATION_02/1 -> bus_creator/4  "SRR_FR_CAN_DET_ELEVATION_02"
  SRR_FR_CAN_DET_SUPER_RES_TARGET_02/1 -> bus_creator/5  "SRR_FR_CAN_DET_SUPER_RES_TARGET_02"
  SRR_FR_CAN_DET_AMPLITUDE_02/1 -> bus_creator/6  "SRR_FR_CAN_DET_AMPLITUDE_02"
  SRR_FR_CAN_DET_VALID_LEVEL_02/1 -> bus_creator/7  "SRR_FR_CAN_DET_VALID_LEVEL_02"

== system P702_NI_SoftECU/Output/Subsystem2/To_NI_HIL/SRR_R/FR_SOD/SRR_FR_003 ==
  SRR_FR_CAN_DET_AMPLITUDE_03 : Constant  Value=0
  SRR_FR_CAN_DET_AZIMUTH_03 : Constant  Value=0
  SRR_FR_CAN_DET_ELEVATION_03 : Constant  Value=0
  SRR_FR_CAN_DET_RANGE_03 : Constant  Value=0
  SRR_FR_CAN_DET_RANGE_RATE_03 : Constant  Value=0
  SRR_FR_CAN_DET_SUPER_RES_TARGET_03 : Constant  Value=0
  SRR_FR_CAN_DET_VALID_LEVEL_03 : Constant  Value=0
  bus_creator : BusCreator  Inputs=7
  out_port : Outport
  wires:
  bus_creator/1 -> out_port/1  "Subsystem2"
  SRR_FR_CAN_DET_RANGE_03/1 -> bus_creator/1  "SRR_FR_CAN_DET_RANGE_03"
  SRR_FR_CAN_DET_RANGE_RATE_03/1 -> bus_creator/2  "SRR_FR_CAN_DET_RANGE_RATE_03"
  SRR_FR_CAN_DET_AZIMUTH_03/1 -> bus_creator/3  "SRR_FR_CAN_DET_AZIMUTH_03"
  SRR_FR_CAN_DET_ELEVATION_03/1 -> bus_creator/4  "SRR_FR_CAN_DET_ELEVATION_03"
  SRR_FR_CAN_DET_SUPER_RES_TARGET_03/1 -> bus_creator/5  "SRR_FR_CAN_DET_SUPER_RES_TARGET_03"
  SRR_FR_CAN_DET_AMPLITUDE_03/1 -> bus_creator/6  "SRR_FR_CAN_DET_AMPLITUDE_03"
  SRR_FR_CAN_DET_VALID_LEVEL_03/1 -> bus_creator/7  "SRR_FR_CAN_DET_VALID_LEVEL_03"

== system P702_NI_SoftECU/Output/Subsystem2/To_NI_HIL/SRR_R/RR_SOD/SRR_RR_001 ==
  SRR_RR_CAN_DET_AMPLITUDE_01 : Constant  Value=0
  SRR_RR_CAN_DET_AZIMUTH_01 : Constant  Value=0
  SRR_RR_CAN_DET_ELEVATION_01 : Constant  Value=0
  SRR_RR_CAN_DET_RANGE_01 : Constant  Value=0
  SRR_RR_CAN_DET_RANGE_RATE_01 : Constant  Value=0
  SRR_RR_CAN_DET_SUPER_RES_TARGET_01 : Constant  Value=0
  SRR_RR_CAN_DET_VALID_LEVEL_01 : Constant  Value=0
  bus_creator : BusCreator  Inputs=7
  out_port : Outport
  wires:
  bus_creator/1 -> out_port/1  "Subsystem2"
  SRR_RR_CAN_DET_RANGE_01/1 -> bus_creator/1  "SRR_RR_CAN_DET_RANGE_01"
  SRR_RR_CAN_DET_RANGE_RATE_01/1 -> bus_creator/2  "SRR_RR_CAN_DET_RANGE_RATE_01"
  SRR_RR_CAN_DET_AZIMUTH_01/1 -> bus_creator/3  "SRR_RR_CAN_DET_AZIMUTH_01"
  SRR_RR_CAN_DET_ELEVATION_01/1 -> bus_creator/4  "SRR_RR_CAN_DET_ELEVATION_01"
  SRR_RR_CAN_DET_SUPER_RES_TARGET_01/1 -> bus_creator/5  "SRR_RR_CAN_DET_SUPER_RES_TARGET_01"
  SRR_RR_CAN_DET_AMPLITUDE_01/1 -> bus_creator/6  "SRR_RR_CAN_DET_AMPLITUDE_01"
  SRR_RR_CAN_DET_VALID_LEVEL_01/1 -> bus_creator/7  "SRR_RR_CAN_DET_VALID_LEVEL_01"

== system P702_NI_SoftECU/Output/Subsystem2/To_NI_HIL/SRR_R/RR_SOD/SRR_RR_002 ==
  SRR_RR_CAN_DET_AMPLITUDE_02 : Constant  Value=0
  SRR_RR_CAN_DET_AZIMUTH_02 : Constant  Value=0
  SRR_RR_CAN_DET_ELEVATION_02 : Constant  Value=0
  SRR_RR_CAN_DET_RANGE_02 : Constant  Value=0
  SRR_RR_CAN_DET_RANGE_RATE_02 : Constant  Value=0
  SRR_RR_CAN_DET_SUPER_RES_TARGET_02 : Constant  Value=0
  SRR_RR_CAN_DET_VALID_LEVEL_02 : Constant  Value=0
  bus_creator : BusCreator  Inputs=7
  out_port : Outport
  wires:
  bus_creator/1 -> out_port/1  "Subsystem2"
  SRR_RR_CAN_DET_RANGE_02/1 -> bus_creator/1  "SRR_RR_CAN_DET_RANGE_02"
  SRR_RR_CAN_DET_RANGE_RATE_02/1 -> bus_creator/2  "SRR_RR_CAN_DET_RANGE_RATE_02"
  SRR_RR_CAN_DET_AZIMUTH_02/1 -> bus_creator/3  "SRR_RR_CAN_DET_AZIMUTH_02"
  SRR_RR_CAN_DET_ELEVATION_02/1 -> bus_creator/4  "SRR_RR_CAN_DET_ELEVATION_02"
  SRR_RR_CAN_DET_SUPER_RES_TARGET_02/1 -> bus_creator/5  "SRR_RR_CAN_DET_SUPER_RES_TARGET_02"
  SRR_RR_CAN_DET_AMPLITUDE_02/1 -> bus_creator/6  "SRR_RR_CAN_DET_AMPLITUDE_02"
  SRR_RR_CAN_DET_VALID_LEVEL_02/1 -> bus_creator/7  "SRR_RR_CAN_DET_VALID_LEVEL_02"

== system P702_NI_SoftECU/Output/Subsystem2/To_NI_HIL/SRR_R/RR_SOD/SRR_RR_003 ==
  SRR_RR_CAN_DET_AMPLITUDE_03 : Constant  Value=0
  SRR_RR_CAN_DET_AZIMUTH_03 : Constant  Value=0
  SRR_RR_CAN_DET_ELEVATION_03 : Constant  Value=0
  SRR_RR_CAN_DET_RANGE_03 : Constant  Value=0
  SRR_RR_CAN_DET_RANGE_RATE_03 : Constant  Value=0
  SRR_RR_CAN_DET_SUPER_RES_TARGET_03 : Constant  Value=0
  SRR_RR_CAN_DET_VALID_LEVEL_03 : Constant  Value=0
  bus_creator : BusCreator  Inputs=7
  out_port : Outport
  wires:
  bus_creator/1 -> out_port/1  "Subsystem2"
  SRR_RR_CAN_DET_RANGE_03/1 -> bus_creator/1  "SRR_RR_CAN_DET_RANGE_03"
  SRR_RR_CAN_DET_RANGE_RATE_03/1 -> bus_creator/2  "SRR_RR_CAN_DET_RANGE_RATE_03"
  SRR_RR_CAN_DET_AZIMUTH_03/1 -> bus_creator/3  "SRR_RR_CAN_DET_AZIMUTH_03"
  SRR_RR_CAN_DET_ELEVATION_03/1 -> bus_creator/4  "SRR_RR_CAN_DET_ELEVATION_03"
  SRR_RR_CAN_DET_SUPER_RES_TARGET_03/1 -> bus_creator/5  "SRR_RR_CAN_DET_SUPER_RES_TARGET_03"
  SRR_RR_CAN_DET_AMPLITUDE_03/1 -> bus_creator/6  "SRR_RR_CAN_DET_AMPLITUDE_03"
  SRR_RR_CAN_DET_VALID_LEVEL_03/1 -> bus_creator/7  "SRR_RR_CAN_DET_VALID_LEVEL_03"

== system P702_NI_SoftECU/Output/Subsystem2/To_NI_HIL/Soft_MRR/MRR_Detection/MRR_Detection_001 ==
  CAN_DET_AMPLITUDE_01 : Constant  Value=0
  CAN_DET_AZIMUTH_01 : Constant  Value=0
  CAN_DET_RANGE_01 : Constant  Value=0
  CAN_DET_RANGE_RATE_01 : Constant  Value=0
  CAN_DET_VALID_LEVEL_01 : Constant  Value=0
  bus_creator : BusCreator  Inputs=5
  out_port : Outport
  wires:
  bus_creator/1 -> out_port/1  "Subsystem2"
  CAN_DET_RANGE_01/1 -> bus_creator/1  "CAN_DET_RANGE_01"
  CAN_DET_RANGE_RATE_01/1 -> bus_creator/2  "CAN_DET_RANGE_RATE_01"
  CAN_DET_AZIMUTH_01/1 -> bus_creator/3  "CAN_DET_AZIMUTH_01"
  CAN_DET_VALID_LEVEL_01/1 -> bus_creator/4  "CAN_DET_VALID_LEVEL_01"
  CAN_DET_AMPLITUDE_01/1 -> bus_creator/5  "CAN_DET_AMPLITUDE_01"

== system P702_NI_SoftECU/Output/Subsystem2/To_NI_HIL/Soft_MRR/MRR_Detection/MRR_Detection_002 ==
  CAN_DET_AMPLITUDE_02 : Constant  Value=0
  CAN_DET_AZIMUTH_02 : Constant  Value=0
  CAN_DET_RANGE_02 : Constant  Value=0
  CAN_DET_RANGE_RATE_02 : Constant  Value=0
  CAN_DET_VALID_LEVEL_02 : Constant  Value=0
  bus_creator : BusCreator  Inputs=5
  out_port : Outport
  wires:
  bus_creator/1 -> out_port/1  "Subsystem2"
  CAN_DET_RANGE_02/1 -> bus_creator/1  "CAN_DET_RANGE_02"
  CAN_DET_RANGE_RATE_02/1 -> bus_creator/2  "CAN_DET_RANGE_RATE_02"
  CAN_DET_AZIMUTH_02/1 -> bus_creator/3  "CAN_DET_AZIMUTH_02"
  CAN_DET_VALID_LEVEL_02/1 -> bus_creator/4  "CAN_DET_VALID_LEVEL_02"
  CAN_DET_AMPLITUDE_02/1 -> bus_creator/5  "CAN_DET_AMPLITUDE_02"

== system P702_NI_SoftECU/Output/Subsystem2/To_NI_HIL/Soft_MRR/MRR_Detection/MRR_Detection_003 ==
  CAN_DET_AMPLITUDE_03 : Constant  Value=0
  CAN_DET_AZIMUTH_03 : Constant  Value=0
  CAN_DET_RANGE_03 : Constant  Value=0
  CAN_DET_RANGE_RATE_03 : Constant  Value=0
  CAN_DET_VALID_LEVEL_03 : Constant  Value=0
  bus_creator : BusCreator  Inputs=5
  out_port : Outport
  wires:
  bus_creator/1 -> out_port/1  "Subsystem2"
  CAN_DET_RANGE_03/1 -> bus_creator/1  "CAN_DET_RANGE_03"
  CAN_DET_RANGE_RATE_03/1 -> bus_creator/2  "CAN_DET_RANGE_RATE_03"
  CAN_DET_AZIMUTH_03/1 -> bus_creator/3  "CAN_DET_AZIMUTH_03"
  CAN_DET_VALID_LEVEL_03/1 -> bus_creator/4  "CAN_DET_VALID_LEVEL_03"
  CAN_DET_AMPLITUDE_03/1 -> bus_creator/5  "CAN_DET_AMPLITUDE_03"

== system P702_NI_SoftECU/SoftECU/PCM/Logic1/Key/PowerStates/Subsystem1 ==
  No_KeyPostn : Inport
  BatterySwitch_B : Inport  Port=2
  BattOff : Constant  Value=0
  Compare To Zero : simulink/Logic and Bit Operations/Compare To Zero  relop=>=  OutDataTypeStr=uint8  ZeroCross=off
  IsTE15 : simulink/Logic and Bit Operations/Compare To Constant  relop===  const=2  OutDataTypeStr=boolean  ZeroCross=off
  IsTE50 : simulink/Logic and Bit Operations/Compare To Constant  relop===  const=3  OutDataTypeStr=boolean  ZeroCross=off
  IsTE75 : simulink/Logic and Bit Operations/Compare To Constant  relop===  const=1  OutDataTypeStr=uint8  ZeroCross=off
  Logical Operator : Logic  AllPortsSameDT=off  OutDataTypeStr=boolean
  Logical Operator1 : Logic  Operator=OR  AllPortsSameDT=off  OutDataTypeStr=boolean
  Logical Operator2 : Logic  Operator=OR  AllPortsSameDT=off  OutDataTypeStr=boolean
  Switch : Switch  Criteria=u2 > Threshold
  Te50_B : Outport
  Te15_B : Outport  Port=2
  Te75_B : Outport  Port=3
  KeyIn_B : Outport  Port=4
  wires:
  Logical Operator1/1 -> Te75_B/1
  IsTE75/1 -> Logical Operator1/2
  Logical Operator2/1 -> Te15_B/1
  Switch/1 -> IsTE75/1, IsTE50/1, IsTE15/1
  BattOff/1 -> Switch/3
  No_KeyPostn/1 -> Switch/1, Compare To Zero/1
  BatterySwitch_B/1 -> Switch/2, Logical Operator/2
  IsTE50/1 -> Te50_B/1, Logical Operator2/1
  IsTE15/1 -> Logical Operator1/1, Logical Operator2/2
  Compare To Zero/1 -> Logical Operator/1
  Logical Operator/1 -> KeyIn_B/1

== system P702_NI_SoftECU/SoftECU/PCM/Mapping/EngineData_7/FuelFlw_Vl_Dsply/Count ==
  Stepsize : Inport
  MaxValue : Inport  Port=2
  Reset : Inport  Port=3
  Enable : EnablePort
  Gain : Gain  Gain=1000
  Integrator1 : Integrator  ExternalReset=rising  InitialConditionSource=external
  Math Function : Math  Operator=mod  SaturateOnIntegerOverflow=on
  Product : Product  RndMeth=Zero
  Relational Operator : RelationalOperator  Operator=<  OutDataTypeStr=boolean  RndMeth=Nearest
  Sum1 : Sum  Inputs=|++
  Xo1 : Constant  Value=0
  offset : Constant  Value=0
  OdoCount : Outport
  OverallCount : Outport  Port=2
  wires:
  Product/1 -> OdoCount/1
  Relational Operator/1 -> Product/2
  Sum1/1 -> Math Function/2
  MaxValue/1 -> Relational Operator/2, Sum1/1
  offset/1 -> Sum1/2
  Math Function/1 -> Product/1, Relational Operator/1
  Xo1/1 -> Integrator1/3
  Integrator1/1 -> Math Function/1, OverallCount/1
  Reset/1 -> Integrator1/2
  Stepsize/1 -> Gain/1
  Gain/1 -> Integrator1/1

== system P702_NI_SoftECU/SoftECU/PCM/Mapping/EngineData_7/FuelFlw_Vl_Dsply/Timer ==
  Stepsize : Inport
  Runtime : Inport  Port=2
  Reset : Inport  Port=3
  Enable : EnablePort
  Data Type Conversion : DataTypeConversion
  Enabled Subsystem : Subsystem  TreatAsAtomicUnit=on
  Gain : Gain
  Integrator : Integrator  ExternalReset=rising  InitialConditionSource=external
  Memory : Memory
  Memory1 : Memory
  Relational Operator : RelationalOperator  Operator=<=  OutDataTypeStr=boolean  RndMeth=Nearest
  Xo : Constant  Value=0
  Active : Outport
  ElapsedTime : Outport  Port=2
  wires:
  Memory1/1 -> Enabled Subsystem/Enable
  Enabled Subsystem/1(Out1) -> ElapsedTime/1
  Runtime/1 -> Relational Operator/2
  Xo/1 -> Integrator/3
  Data Type Conversion/1 -> Integrator/2
  Relational Operator/1 -> Memory1/1, Active/1
  Reset/1 -> Data Type Conversion/1
  Memory/1 -> Enabled Subsystem/1(In1), Relational Operator/1
  Stepsize/1 -> Gain/1
  Gain/1 -> Integrator/1
  Integrator/1 -> Memory/1

== system P702_NI_SoftECU/SoftECU/PCM/Mapping/EngineData_7/ODoCount/Count ==
  Stepsize : Inport
  MaxValue : Inport  Port=2
  Reset : Inport  Port=3
  Enable : EnablePort
  Gain : Gain  Gain=1000
  Integrator1 : Integrator  ExternalReset=rising  InitialConditionSource=external
  Math Function : Math  Operator=mod  SaturateOnIntegerOverflow=on
  Product : Product  RndMeth=Zero
  Relational Operator : RelationalOperator  Operator=<  OutDataTypeStr=boolean  RndMeth=Nearest
  Sum1 : Sum  Inputs=|++
  Xo1 : Constant  Value=0
  offset : Constant
  OdoCount : Outport
  OverallCount : Outport  Port=2
  wires:
  Product/1 -> OdoCount/1
  Relational Operator/1 -> Product/2
  Sum1/1 -> Math Function/2
  MaxValue/1 -> Relational Operator/2, Sum1/1
  offset/1 -> Sum1/2
  Math Function/1 -> Product/1, Relational Operator/1
  Xo1/1 -> Integrator1/3
  Integrator1/1 -> Math Function/1, OverallCount/1
  Reset/1 -> Integrator1/2
  Stepsize/1 -> Gain/1
  Gain/1 -> Integrator1/1

== system P702_NI_SoftECU/SoftECU/PCM/Mapping/EngineData_7/ODoCount/Timer ==
  Stepsize : Inport
  Runtime : Inport  Port=2
  Reset : Inport  Port=3
  Enable : EnablePort
  Data Type Conversion : DataTypeConversion
  Enabled Subsystem : Subsystem  TreatAsAtomicUnit=on
  Gain : Gain
  Integrator : Integrator  ExternalReset=rising  InitialConditionSource=external
  Memory : Memory
  Memory1 : Memory
  Relational Operator : RelationalOperator  Operator=<=  OutDataTypeStr=boolean  RndMeth=Nearest
  Xo : Constant  Value=0
  Active : Outport
  ElapsedTime : Outport  Port=2
  wires:
  Memory1/1 -> Enabled Subsystem/Enable
  Enabled Subsystem/1(Out1) -> ElapsedTime/1
  Runtime/1 -> Relational Operator/2
  Xo/1 -> Integrator/3
  Data Type Conversion/1 -> Integrator/2
  Relational Operator/1 -> Memory1/1, Active/1
  Reset/1 -> Data Type Conversion/1
  Memory/1 -> Enabled Subsystem/1(In1), Relational Operator/1
  Stepsize/1 -> Gain/1
  Gain/1 -> Integrator/1
  Integrator/1 -> Memory/1

== system P702_NI_SoftECU/SoftECU/SCCM/Logic/Map_Inputs/Maneuver/pos_edge_detection ==
  In1 : Inport
  Memory : Memory
  Relational Operator : RelationalOperator  Operator=>  OutDataTypeStr=boolean  RndMeth=Nearest
  Out1 : Outport
  wires:
  In1/1 -> Relational Operator/1, Memory/1
  Relational Operator/1 -> Out1/1
  Memory/1 -> Relational Operator/2

== system P702_NI_SoftECU/SoftECU/SCCM/Logic/Map_Inputs/Maneuver/pos_edge_detection1 ==
  In1 : Inport
  Memory : Memory
  Relational Operator : RelationalOperator  Operator=>  OutDataTypeStr=boolean  RndMeth=Nearest
  Out1 : Outport
  wires:
  Memory/1 -> Relational Operator/2
  Relational Operator/1 -> Out1/1
  In1/1 -> Memory/1, Relational Operator/1

== system P702_NI_SoftECU/SoftECU/SCCM/Logic/Map_Inputs/Maneuver/pos_edge_detection2 ==
  In1 : Inport
  Memory : Memory
  Relational Operator : RelationalOperator  Operator=>  OutDataTypeStr=boolean  RndMeth=Nearest
  Out1 : Outport
  wires:
  In1/1 -> Relational Operator/1, Memory/1
  Relational Operator/1 -> Out1/1
  Memory/1 -> Relational Operator/2

== system P702_NI_SoftECU/SoftECU/SCCM/Logic/Map_Inputs/Maneuver/pos_edge_detection3 ==
  In1 : Inport
  Memory : Memory
  Relational Operator : RelationalOperator  Operator=>  OutDataTypeStr=boolean  RndMeth=Nearest
  Out1 : Outport
  wires:
  Memory/1 -> Relational Operator/2
  Relational Operator/1 -> Out1/1
  In1/1 -> Memory/1, Relational Operator/1

== system P702_NI_SoftECU/SoftECU/SRR_L/FrontLeft_SOD/SRR_FL_001/Subsystem/random_factor ==
  Range : Inport
  1-D Lookup Table : Lookup_n-D  NumberOfTableDimensions=1  BreakpointsForDimension1=[-10 10 20 40 80 1000]  Table="[1   1   1.2  2   3 3]"  InternalRulePriority=Speed  RndMeth=Simplest  InputSameDT=on
  Gain : Gain
  Product3 : Product  Inputs=3
  Random Number : RandomNumber  Variance=0.3  SampleTime=0.1
  Saturation : Saturate  UpperLimit=0.3  LowerLimit=-0.3
  Rand_Error : Outport
  wires:
  [Random_Status] -> Product3/3
  Saturation/1 -> Gain/1
  Product3/1 -> Rand_Error/1
  Range/1 -> 1-D Lookup Table/1
  1-D Lookup Table/1 -> Product3/1
  Gain/1 -> Product3/2
  Random Number/1 -> Saturation/1

== system P702_NI_SoftECU/SoftECU/SRR_L/FrontLeft_SOD/SRR_FL_001/Subsystem/random_factor1 ==
  Range : Inport
  1-D Lookup Table : Lookup_n-D  NumberOfTableDimensions=1  BreakpointsForDimension1=[-10 10 20 40 80 1000]  Table="[1   1   1.2  2   3 3]"  InternalRulePriority=Speed  RndMeth=Simplest  InputSameDT=on
  Gain : Gain
  Product3 : Product  Inputs=3
  Random Number : RandomNumber  Variance=0.3  SampleTime=0.1
  Saturation : Saturate  UpperLimit=0.3  LowerLimit=-0.3
  Rand_Error : Outport
  wires:
  [Random_Status] -> Product3/3
  Saturation/1 -> Gain/1
  Product3/1 -> Rand_Error/1
  Range/1 -> 1-D Lookup Table/1
  1-D Lookup Table/1 -> Product3/1
  Gain/1 -> Product3/2
  Random Number/1 -> Saturation/1

== system P702_NI_SoftECU/SoftECU/SRR_L/FrontLeft_SOD/SRR_FL_002/Subsystem/random_factor ==
  Range : Inport
  1-D Lookup Table : Lookup_n-D  NumberOfTableDimensions=1  BreakpointsForDimension1=[-10 10 20 40 80 1000]  Table="[1   1   1.2  2   3 3]"  InternalRulePriority=Speed  RndMeth=Simplest  InputSameDT=on
  Gain : Gain
  Product3 : Product  Inputs=3
  Random Number : RandomNumber  Variance=0.3  SampleTime=0.1
  Saturation : Saturate  UpperLimit=0.3  LowerLimit=-0.3
  Rand_Error : Outport
  wires:
  Random Number/1 -> Saturation/1
  Gain/1 -> Product3/2
  1-D Lookup Table/1 -> Product3/1
  Range/1 -> 1-D Lookup Table/1
  Product3/1 -> Rand_Error/1
  Saturation/1 -> Gain/1
  [Random_Status] -> Product3/3

== system P702_NI_SoftECU/SoftECU/SRR_L/FrontLeft_SOD/SRR_FL_002/Subsystem/random_factor1 ==
  Range : Inport
  1-D Lookup Table : Lookup_n-D  NumberOfTableDimensions=1  BreakpointsForDimension1=[-10 10 20 40 80 1000]  Table="[1   1   1.2  2   3 3]"  InternalRulePriority=Speed  RndMeth=Simplest  InputSameDT=on
  Gain : Gain
  Product3 : Product  Inputs=3
  Random Number : RandomNumber  Variance=0.3  SampleTime=0.1
  Saturation : Saturate  UpperLimit=0.3  LowerLimit=-0.3
  Rand_Error : Outport
  wires:
  Random Number/1 -> Saturation/1
  Gain/1 -> Product3/2
  1-D Lookup Table/1 -> Product3/1
  Range/1 -> 1-D Lookup Table/1
  Product3/1 -> Rand_Error/1
  Saturation/1 -> Gain/1
  [Random_Status] -> Product3/3

== system P702_NI_SoftECU/SoftECU/SRR_L/FrontLeft_SOD/SRR_FL_003/Subsystem/random_factor ==
  Range : Inport
  1-D Lookup Table : Lookup_n-D  NumberOfTableDimensions=1  BreakpointsForDimension1=[-10 10 20 40 80 1000]  Table="[1   1   1.2  2   3 3]"  InternalRulePriority=Speed  RndMeth=Simplest  InputSameDT=on
  Gain : Gain
  Product3 : Product  Inputs=3
  Random Number : RandomNumber  Variance=0.3  SampleTime=0.1
  Saturation : Saturate  UpperLimit=0.3  LowerLimit=-0.3
  Rand_Error : Outport
  wires:
  [Random_Status] -> Product3/3
  Saturation/1 -> Gain/1
  Product3/1 -> Rand_Error/1
  Range/1 -> 1-D Lookup Table/1
  1-D Lookup Table/1 -> Product3/1
  Gain/1 -> Product3/2
  Random Number/1 -> Saturation/1

== system P702_NI_SoftECU/SoftECU/SRR_L/FrontLeft_SOD/SRR_FL_003/Subsystem/random_factor1 ==
  Range : Inport
  1-D Lookup Table : Lookup_n-D  NumberOfTableDimensions=1  BreakpointsForDimension1=[-10 10 20 40 80 1000]  Table="[1   1   1.2  2   3 3]"  InternalRulePriority=Speed  RndMeth=Simplest  InputSameDT=on
  Gain : Gain
  Product3 : Product  Inputs=3
  Random Number : RandomNumber  Variance=0.3  SampleTime=0.1
  Saturation : Saturate  UpperLimit=0.3  LowerLimit=-0.3
  Rand_Error : Outport
  wires:
  [Random_Status] -> Product3/3
  Saturation/1 -> Gain/1
  Product3/1 -> Rand_Error/1
  Range/1 -> 1-D Lookup Table/1
  1-D Lookup Table/1 -> Product3/1
  Gain/1 -> Product3/2
  Random Number/1 -> Saturation/1

== system P702_NI_SoftECU/SoftECU/SRR_L/RearLeft_SOD/SRR_RL_001 /Subsystem/random_factor ==
  Range : Inport
  1-D Lookup Table : Lookup_n-D  NumberOfTableDimensions=1  BreakpointsForDimension1=[-10 10 20 40 80 1000]  Table="[1   1   1.2  2   3 3]"  InternalRulePriority=Speed  RndMeth=Simplest  InputSameDT=on
  Gain : Gain
  Product3 : Product  Inputs=3
  Random Number : RandomNumber  Variance=0.3  SampleTime=0.1
  Saturation : Saturate  UpperLimit=0.3  LowerLimit=-0.3
  Rand_Error : Outport
  wires:
  Random Number/1 -> Saturation/1
  Gain/1 -> Product3/2
  1-D Lookup Table/1 -> Product3/1
  Range/1 -> 1-D Lookup Table/1
  Product3/1 -> Rand_Error/1
  Saturation/1 -> Gain/1
  [Random_Status] -> Product3/3

== system P702_NI_SoftECU/SoftECU/SRR_L/RearLeft_SOD/SRR_RL_001 /Subsystem/random_factor1 ==
  Range : Inport
  1-D Lookup Table : Lookup_n-D  NumberOfTableDimensions=1  BreakpointsForDimension1=[-10 10 20 40 80 1000]  Table="[1   1   1.2  2   3 3]"  InternalRulePriority=Speed  RndMeth=Simplest  InputSameDT=on
  Gain : Gain
  Product3 : Product  Inputs=3
  Random Number : RandomNumber  Variance=0.3  SampleTime=0.1
  Saturation : Saturate  UpperLimit=0.3  LowerLimit=-0.3
  Rand_Error : Outport
  wires:
  Random Number/1 -> Saturation/1
  Gain/1 -> Product3/2
  1-D Lookup Table/1 -> Product3/1
  Range/1 -> 1-D Lookup Table/1
  Product3/1 -> Rand_Error/1
  Saturation/1 -> Gain/1
  [Random_Status] -> Product3/3
